simulink model "EngineComponent1"  (R2021b)
settings: Solver=VariableStepAuto  StartTime=0.0  StopTime=30.0  RelTol=1e-3
libraries: simulink x1
settings Model: Creator=김태진  LastModifiedBy=김태진
settings SolverCC: AlgebraicLoopSolver=TrustRegion
settings DebuggingCC: SFMachineParentedDataDiag=warning

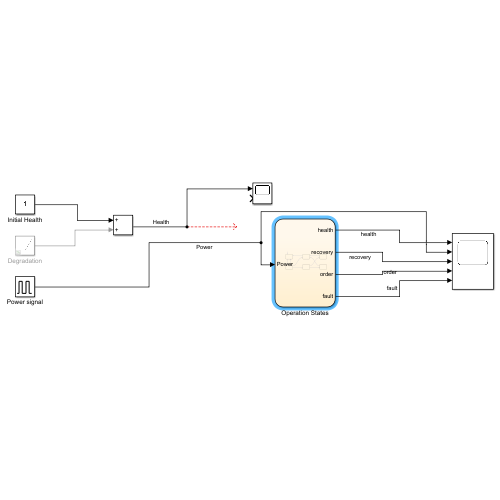
[thumbnail: Simulink's stored preview of the top-level diagram]
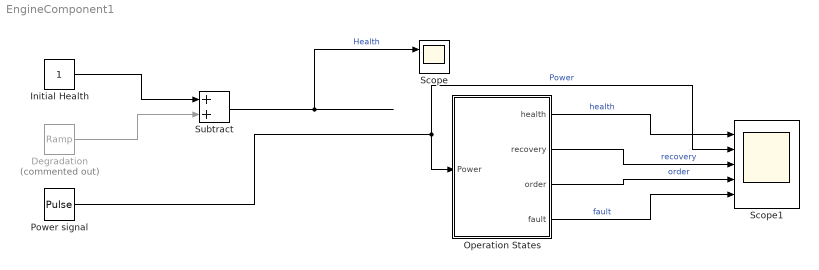
== system EngineComponent1 ==
  Degradation : simulink/Sources/Ramp  Commented=on  slope=-0.1  start=0  InitialOutput=0
  Initial Health : Constant
  Operation States : Stateflow chart  TreatAsAtomicUnit=on
  Power signal : DiscretePulseGenerator  PulseType=Time based  Period=10  PulseWidth=50
  Scope : Scope  NumInputPorts=2
  Scope1 : Scope  NumInputPorts=5
  Subtract : Sum
  wires:
  Initial Health/1 -> Subtract/1
  Degradation/1 -> Subtract/2
  Subtract/1 -> Scope/1  "Health"
  Power signal/1 -> Scope1/2, Operation States/1(Power)  "Power"
  Operation States/1(health) -> Scope1/1  "health"
  Operation States/2(recovery) -> Scope1/3  "recovery"
  Operation States/3(order) -> Scope1/4  "order"
  Operation States/4(fault) -> Scope1/5  "fault"

== stateflow chart EngineComponent1/Operation States ==
  note: Inspection
  note: Maintenance
  state On
    during:
    health = health - 0.02;
    useTime = useTime + 1;
  state Normal
  state Recovery
    entry:
    recovery = 1;
    counter = 0;
    during:
    counter = counter +1;
    exit:
    recovery = 0;
    health = 1;
  note: Maintenance
  state Off
  state UseTimeMaintenance
  state Replacement
  state Diagnosis
  state Fault
    entry:
    fault = 1;
    exit:
    fault = 0;
  note: Need checkInventory() method
  state Order
    entry:
    order = 1;
    counter = 0;
    during:
    counter = counter +1;
    exit:
    order = 0;
    health = 1;
  state CalendarMaintenance [commented out]
  note: Need Global Variable "calendarTime"
  state PredictiveMaintenance
  (default) -> On : {health = 1; useTime=0;}
  Recovery -> Normal : [counter > 5]
  Normal -> On : [Power == 1]
  Order -> Normal : [counter > 5]
  Fault -> Recovery [order 1] : [false]
  Diagnosis -> Normal [order 2] : [health > 0.8]
  On -> Off : [Power == 0]
  Off -> UseTimeMaintenance
  UseTimeMaintenance -> Replacement
  Diagnosis -> Fault [order 1] : [health <= 0.8]
  Fault -> Order [order 2]
  data: Power input; health output; counter local; recovery output; order output; fault output; useTime local
